simulink model "Final_Simulink_Model_assignment_2"  (R2022b)
settings: Solver=FixedStepAuto  StartTime=0.0  StopTime=inf  FixedStep=1e-3  RelTol=1e-3  EnableMultiTasking=on
undefined symbols (not defined in the file): A0, A1, ATR_PULSE_WIDTH, ATR_PUSLE_WIDTH, D0, D1, D10, D11, D12, D13, D2, D3, D4, D5, D6, D7, D8, D9, LRL, magnitude, PTA0, PTA1, PTA2, PTB2, PTB23, PTB3, PTB9, PTC16, PTC17, PTC2, PTC3, PTC4, PTD0, PTD1, PTD2, PTD3, REF_PERIOD, REF_PREIOD, VENT_PULSE_WIDTH
libraries: frdmk64flib x30, etargetslib x9, dspstat3 x1
(part 2 of 2)

== stateflow chart Final_Simulink_Model_assignment_2/Requirements Table1 ==
  (default) -> (junction 1073743363)
  (junction 1073743363) -> (junction 1073743364) : {
      | % SF_REQ_REV_07
      | }
  (junction 1073743364) -> (junction 1073743366) : {
      | % HEADER_ASSIGNMENTS
      |
      | }
  (junction 1073743366) -> (junction 1073743368) : {
      | % START_A_4
      | }
  (junction 1073743368) -> (junction 1073743370) : {
      | }
  (junction 1073743370) -> (junction 1073743372)
  (junction 1073743372) -> (junction 1073743374) : {
      | }
  (junction 1073743374) -> (junction 1073743376) : {
      | % END_A_4
      | }
  (junction 1073743376) -> (junction 1073743378) : {
      | % START_R_1
      | }
  (junction 1073743378) -> (junction 1073743380) : {
      | }
  (junction 1073743380) -> (junction 1073743382)
  (junction 1073743382) -> (junction 1073743384) [order 1] : [(((Mode) == (1)))]
  (junction 1073743382) -> (junction 1073743426) [order 2]
  (junction 1073743384) -> (junction 1073743386) : {
      |
      |
      | }
  (junction 1073743386) -> (junction 1073743388) : {
      | }
  (junction 1073743388) -> (junction 1073743390) : {
      | % START_R_7
      | }
  (junction 1073743390) -> (junction 1073743392) : {
      | }
  (junction 1073743392) -> (junction 1073743394)
  (junction 1073743394) -> (junction 1073743396) [order 1] : [duration((((State) == (1)))) >= 60000/LRL - ATR_PULSE_WIDTH]
  (junction 1073743394) -> (junction 1073743402) [order 2]
  (junction 1073743396) -> (junction 1073743398) : {
      | reqtable_postcondition((((ATR_PACE_CTRL) == (1))) && (((ATR_GND_CTRL) == (0))) && (((PACE_CHARGE_CTRL) == (0))) && (((PACE_GND_CTRL) == (1))), 'R:1.1');
      |
      |
      | }
  (junction 1073743398) -> (junction 1073743400) : {
      | }
  (junction 1073743400) -> (junction 1073743402)
  (junction 1073743402) -> (junction 1073743404)
  (junction 1073743404) -> (junction 1073743406) : {
      | % END_R_7
      | }
  (junction 1073743406) -> (junction 1073743408) : {
      | % START_R_10
      | }
  (junction 1073743408) -> (junction 1073743410) : {
      | }
  (junction 1073743410) -> (junction 1073743412)
  (junction 1073743412) -> (junction 1073743414) [order 1] : [duration((((State) == (2)))) >= ATR_PULSE_WIDTH]
  (junction 1073743412) -> (junction 1073743420) [order 2]
  (junction 1073743414) -> (junction 1073743416) : {
      | reqtable_postcondition((((ATR_PACE_CTRL) == (0))) && (((ATR_GND_CTRL) == (1))) && (((PACE_CHARGE_CTRL) == (1))) && (((PACE_GND_CTRL) == (1))), 'R:1.2');
      |
      |
      | }
  (junction 1073743416) -> (junction 1073743418) : {
      | }
  (junction 1073743418) -> (junction 1073743420)
  (junction 1073743420) -> (junction 1073743422)
  (junction 1073743422) -> (junction 1073743424) : {
      | % END_R_10
      | }
  (junction 1073743424) -> (junction 1073743426)
  (junction 1073743426) -> (junction 1073743428)
  (junction 1073743428) -> (junction 1073743672) : {
      | % END_R_1
      | }
  (junction 1073743672) -> (junction 1073743432) : {
      | % START_R_13
      | }
  (junction 1073743432) -> (junction 1073743434) : {
      | }
  (junction 1073743434) -> (junction 1073743436)
  (junction 1073743436) -> (junction 1073743438) [order 1] : [(((Mode) == (2)))]
  (junction 1073743436) -> (junction 1073743480) [order 2]
  (junction 1073743438) -> (junction 1073743440) : {
      |
      |
      | }
  (junction 1073743440) -> (junction 1073743442) : {
      | }
  (junction 1073743442) -> (junction 1073743444) : {
      | % START_R_16
      | }
  (junction 1073743444) -> (junction 1073743446) : {
      | }
  (junction 1073743446) -> (junction 1073743448)
  (junction 1073743448) -> (junction 1073743450) [order 1] : [duration((((State) == (1)))) >= 60000/LRL - VENT_PULSE_WIDTH]
  (junction 1073743448) -> (junction 1073743456) [order 2]
  (junction 1073743450) -> (junction 1073743452) : {
      | reqtable_postcondition((((PACE_CHARGE_CTRL) == (0))) && (((PACE_GND_CTRL) == (1))) && (((VENT_PACE_CTRL) == (1))) && (((VENT_GND_CTRL) == (0))), 'R:2.1');
      |
      |
      | }
  (junction 1073743452) -> (junction 1073743454) : {
      | }
  (junction 1073743454) -> (junction 1073743456)
  (junction 1073743456) -> (junction 1073743458)
  (junction 1073743458) -> (junction 1073743460) : {
      | % END_R_16
      | }
  (junction 1073743460) -> (junction 1073743462) : {
      | % START_R_19
      | }
  (junction 1073743462) -> (junction 1073743464) : {
      | }
  (junction 1073743464) -> (junction 1073743466)
  (junction 1073743466) -> (junction 1073743468) [order 1] : [duration((((State) == (2)))) >= VENT_PULSE_WIDTH]
  (junction 1073743466) -> (junction 1073743474) [order 2]
  (junction 1073743468) -> (junction 1073743470) : {
      | reqtable_postcondition((((PACE_CHARGE_CTRL) == (1))) && (((PACE_GND_CTRL) == (1))) && (((VENT_PACE_CTRL) == (0))) && (((VENT_GND_CTRL) == (1))), 'R:2.2');
      |
      |
      | }
  (junction 1073743470) -> (junction 1073743472) : {
      | }
  (junction 1073743472) -> (junction 1073743474)
  (junction 1073743474) -> (junction 1073743476)
  (junction 1073743476) -> (junction 1073743478) : {
      | % END_R_19
      | }
  (junction 1073743478) -> (junction 1073743480)
  (junction 1073743480) -> (junction 1073743482)
  (junction 1073743482) -> (junction 1073743484) : {
      | % END_R_13
      | }
  (junction 1073743484) -> (junction 1073743486) : {
      | % START_R_22
      | }
  (junction 1073743486) -> (junction 1073743488) : {
      | }
  (junction 1073743488) -> (junction 1073743490)
  (junction 1073743490) -> (junction 1073743492) [order 1] : [(((Mode) == (3)))]
  (junction 1073743490) -> (junction 1073743552) [order 2]
  (junction 1073743492) -> (junction 1073743494) : {
      |
      |
      | }
  (junction 1073743494) -> (junction 1073743496) : {
      | }
  (junction 1073743496) -> (junction 1073743498) : {
      | % START_R_25
      | }
  (junction 1073743498) -> (junction 1073743500) : {
      | }
  (junction 1073743500) -> (junction 1073743502)
  (junction 1073743502) -> (junction 1073743504) [order 1] : [duration((((State) == (1)))) >= 60000/LRL - ATR_PULSE_WIDTH]
  (junction 1073743502) -> (junction 1073743510) [order 2]
  (junction 1073743504) -> (junction 1073743506) : {
      | reqtable_postcondition((((ATR_PACE_CTRL) == (0))) && (((ATR_GND_CTRL) == (1))) && (((PACE_CHARGE_CTRL) == (1))) && (((PACE_GND_CTRL) == (1))) && (((FRONTEND_CTRL) == (1))), 'R:3.1');
      |
      |
      | }
  (junction 1073743506) -> (junction 1073743508) : {
      | }
  (junction 1073743508) -> (junction 1073743510)
  (junction 1073743510) -> (junction 1073743512)
  (junction 1073743512) -> (junction 1073743514) : {
      | % END_R_25
      | }
  (junction 1073743514) -> (junction 1073743516) : {
      | % START_R_28
      | }
  (junction 1073743516) -> (junction 1073743518) : {
      | }
  (junction 1073743518) -> (junction 1073743520)
  (junction 1073743520) -> (junction 1073743522) [order 1] : [duration((((State) == (2)))) >= ATR_PULSE_WIDTH]
  (junction 1073743520) -> (junction 1073743528) [order 2]
  (junction 1073743522) -> (junction 1073743524) : {
      | reqtable_postcondition((((ATR_PACE_CTRL) == (1))) && (((ATR_GND_CTRL) == (0))) && (((PACE_CHARGE_CTRL) == (0))) && (((PACE_GND_CTRL) == (1))), 'R:3.2');
      |
      |
      | }
  (junction 1073743524) -> (junction 1073743526) : {
      | }
  (junction 1073743526) -> (junction 1073743528)
  (junction 1073743528) -> (junction 1073743530)
  (junction 1073743530) -> (junction 1073743532) : {
      | % END_R_28
      | }
  (junction 1073743532) -> (junction 1073743534) : {
      | % START_R_31
      | }
  (junction 1073743534) -> (junction 1073743536) : {
      | }
  (junction 1073743536) -> (junction 1073743538)
  (junction 1073743538) -> (junction 1073743540) [order 1] : [duration((((State) == (3)))) >= REF_PERIOD]
  (junction 1073743538) -> (junction 1073743546) [order 2]
  (junction 1073743540) -> (junction 1073743542) : {
      | reqtable_postcondition((((ATR_PACE_CTRL) == (0))) && (((ATR_GND_CTRL) == (1))) && (((PACE_CHARGE_CTRL) == (0))) && (((PACE_GND_CTRL) == (1))) && (((FRONTEND_CTRL) == (0))), 'R:3.3');
      |
      |
      | }
  (junction 1073743542) -> (junction 1073743544) : {
      | }
  (junction 1073743544) -> (junction 1073743546)
  (junction 1073743546) -> (junction 1073743548)
  (junction 1073743548) -> (junction 1073743550) : {
      | % END_R_31
      | }
  (junction 1073743550) -> (junction 1073743552)
  (junction 1073743552) -> (junction 1073743554)
  (junction 1073743554) -> (junction 1073743556) : {
      | % END_R_22
      | }
  (junction 1073743556) -> (junction 1073743558) : {
      | % START_R_34
      | }
  (junction 1073743558) -> (junction 1073743560) : {
      | }
  (junction 1073743560) -> (junction 1073743562)
  (junction 1073743562) -> (junction 1073743564) [order 1] : [(((Mode) == (4)))]
  (junction 1073743562) -> (junction 1073743624) [order 2]
  (junction 1073743564) -> (junction 1073743566) : {
      |
      |
      | }
  (junction 1073743566) -> (junction 1073743568) : {
      | }
  (junction 1073743568) -> (junction 1073743570) : {
      | % START_R_37
      | }
  (junction 1073743570) -> (junction 1073743572) : {
      | }
  (junction 1073743572) -> (junction 1073743574)
  (junction 1073743574) -> (junction 1073743576) [order 1] : [duration((((State) == (1)))) >= 60000/LRL - VENT_PULSE_WIDTH]
  (junction 1073743574) -> (junction 1073743582) [order 2]
  (junction 1073743576) -> (junction 1073743578) : {
      | reqtable_postcondition((((PACE_CHARGE_CTRL) == (1))) && (((PACE_GND_CTRL) == (1))) && (((VENT_PACE_CTRL) == (0))) && (((VENT_GND_CTRL) == (1))) && (((FRONTEND_CTRL) == (1))), 'R:4.1');
      |
      |
      | }
  (junction 1073743578) -> (junction 1073743580) : {
      | }
  (junction 1073743580) -> (junction 1073743582)
  (junction 1073743582) -> (junction 1073743584)
  (junction 1073743584) -> (junction 1073743586) : {
      | % END_R_37
      | }
  (junction 1073743586) -> (junction 1073743588) : {
      | % START_R_40
      | }
  (junction 1073743588) -> (junction 1073743590) : {
      | }
  (junction 1073743590) -> (junction 1073743592)
  (junction 1073743592) -> (junction 1073743594) [order 1] : [duration((((State) == (2)))) >= VENT_PULSE_WIDTH]
  (junction 1073743592) -> (junction 1073743600) [order 2]
  (junction 1073743594) -> (junction 1073743596) : {
      | reqtable_postcondition((((PACE_CHARGE_CTRL) == (0))) && (((PACE_GND_CTRL) == (1))) && (((VENT_PACE_CTRL) == (1))) && (((VENT_GND_CTRL) == (0))), 'R:4.2');
      |
      |
      | }
  (junction 1073743596) -> (junction 1073743598) : {
      | }
  (junction 1073743598) -> (junction 1073743600)
  (junction 1073743600) -> (junction 1073743602)
  (junction 1073743602) -> (junction 1073743604) : {
      | % END_R_40
      | }
  (junction 1073743604) -> (junction 1073743606) : {
      | % START_R_43
      | }
  (junction 1073743606) -> (junction 1073743608) : {
      | }
  (junction 1073743608) -> (junction 1073743610)
  (junction 1073743610) -> (junction 1073743612) [order 1] : [duration((((State) == (3)))) >= REF_PREIOD]
  (junction 1073743610) -> (junction 1073743618) [order 2]
  (junction 1073743612) -> (junction 1073743614) : {
      | reqtable_postcondition((((PACE_CHARGE_CTRL) == (0))) && (((PACE_GND_CTRL) == (1))) && (((VENT_PACE_CTRL) == (0))) && (((VENT_GND_CTRL) == (1))) && (((FRONTEND_CTRL) == (0))), 'R:4.3');
      |
      |
      | }
  (junction 1073743614) -> (junction 1073743616) : {
      | }
  (junction 1073743616) -> (junction 1073743618)
  (junction 1073743618) -> (junction 1073743620)
  (junction 1073743620) -> (junction 1073743660) : {
      | % END_R_43
      | }
  (junction 1073743660) -> (junction 1073743624)
  (junction 1073743624) -> (junction 1073743626)
  (junction 1073743626) -> (junction 1073743628) : {
      | % END_R_34
      | }
  (junction 1073743628) -> (junction 1073743709) : {
      | % START_R_46
      | }
  (junction 1073743709) -> (junction 1073743711) : {
      | }
  (junction 1073743711) -> (junction 1073743713)
  (junction 1073743713) -> (junction 1073743715) [order 1] : [(((Mode) == (5)))]
  (junction 1073743713) -> (junction 1073743731) [order 2]
  (junction 1073743715) -> (junction 1073743717) : {
      |
      |
      | }
  (junction 1073743717) -> (junction 1073743719) : {
      | }
  (junction 1073743719) -> (junction 1073743786) : {
      | % START_R_49
      | }
  (junction 1073743786) -> (junction 1073743788) : {
      | }
  (junction 1073743788) -> (junction 1073743790)
  (junction 1073743790) -> (junction 1073743792) [order 1] : [duration((((State) == (1)))) >= 60000/Rate-ATR_PULSE_WIDTH]
  (junction 1073743790) -> (junction 1073743798) [order 2]
  (junction 1073743792) -> (junction 1073743794) : {
      | reqtable_postcondition((((ATR_PACE_CTRL) == (1))) && (((ATR_GND_CTRL) == (0))) && (((PACE_CHARGE_CTRL) == (0))) && (((PACE_GND_CTRL) == (1))), 'R:5.1');
      |
      |
      | }
  (junction 1073743794) -> (junction 1073743796) : {
      | }
  (junction 1073743796) -> (junction 1073743798)
  (junction 1073743798) -> (junction 1073743800)
  (junction 1073743800) -> (junction 1073743802) : {
      | % END_R_49
      | }
  (junction 1073743802) -> (junction 1073743807) : {
      | % START_R_52
      | }
  (junction 1073743807) -> (junction 1073743809) : {
      | }
  (junction 1073743809) -> (junction 1073743811)
  (junction 1073743811) -> (junction 1073743813) [order 1] : [duration((((State) == (2)))) >= ATR_PULSE_WIDTH]
  (junction 1073743811) -> (junction 1073743819) [order 2]
  (junction 1073743813) -> (junction 1073743815) : {
      | reqtable_postcondition((((ATR_PACE_CTRL) == (0))) && (((ATR_GND_CTRL) == (1))) && (((PACE_CHARGE_CTRL) == (1))) && (((PACE_GND_CTRL) == (1))), 'R:5.2');
      |
      |
      | }
  (junction 1073743815) -> (junction 1073743817) : {
      | }
  (junction 1073743817) -> (junction 1073743819)
  (junction 1073743819) -> (junction 1073743821)
  (junction 1073743821) -> (junction 1073743823) : {
      | % END_R_52
      | }
  (junction 1073743823) -> (junction 1073743731)
  (junction 1073743731) -> (junction 1073743733)
  (junction 1073743733) -> (junction 1073743735) : {
      | % END_R_46
      | }
  (junction 1073743735) -> (junction 1073743974) : {
      | % START_R_55
      | }
  (junction 1073743974) -> (junction 1073743976) : {
      | }
  (junction 1073743976) -> (junction 1073743978)
  (junction 1073743978) -> (junction 1073743980) [order 1] : [(((Mode) == (6)))]
  (junction 1073743978) -> (junction 1073744022) [order 2]
  (junction 1073743980) -> (junction 1073743982) : {
      |
      |
      | }
  (junction 1073743982) -> (junction 1073743984) : {
      | }
  (junction 1073743984) -> (junction 1073743986) : {
      | % START_R_58
      | }
  (junction 1073743986) -> (junction 1073743988) : {
      | }
  (junction 1073743988) -> (junction 1073743990)
  (junction 1073743990) -> (junction 1073743992) [order 1] : [duration((((State) == (1)))) >= 60000/ Rate- VENT_PULSE_WIDTH]
  (junction 1073743990) -> (junction 1073743998) [order 2]
  (junction 1073743992) -> (junction 1073743994) : {
      | reqtable_postcondition((((PACE_CHARGE_CTRL) == (0))) && (((PACE_GND_CTRL) == (1))) && (((VENT_PACE_CTRL) == (1))) && (((VENT_GND_CTRL) == (0))), 'R:6.1');
      |
      |
      | }
  (junction 1073743994) -> (junction 1073743996) : {
      | }
  (junction 1073743996) -> (junction 1073743998)
  (junction 1073743998) -> (junction 1073744000)
  (junction 1073744000) -> (junction 1073744002) : {
      | % END_R_58
      | }
  (junction 1073744002) -> (junction 1073744004) : {
      | % START_R_61
      | }
  (junction 1073744004) -> (junction 1073744006) : {
      | }
  (junction 1073744006) -> (junction 1073744008)
  (junction 1073744008) -> (junction 1073744010) [order 1] : [duration((((State) == (2)))) >= VENT_PULSE_WIDTH]
  (junction 1073744008) -> (junction 1073744016) [order 2]
  (junction 1073744010) -> (junction 1073744012) : {
      | reqtable_postcondition((((PACE_CHARGE_CTRL) == (1))) && (((PACE_GND_CTRL) == (1))) && (((VENT_PACE_CTRL) == (0))) && (((VENT_GND_CTRL) == (1))), 'R:6.2');
      |
      |
      | }
  (junction 1073744012) -> (junction 1073744014) : {
      | }
  (junction 1073744014) -> (junction 1073744016)
  (junction 1073744016) -> (junction 1073744018)
  (junction 1073744018) -> (junction 1073744020) : {
      | % END_R_61
      | }
  (junction 1073744020) -> (junction 1073744022)
  (junction 1073744022) -> (junction 1073744024)
  (junction 1073744024) -> (junction 1073744026) : {
      | % END_R_55
      | }
  (junction 1073744026) -> (junction 1073744033) : {
      | % START_R_64
      | }
  (junction 1073744033) -> (junction 1073744035) : {
      | }
  (junction 1073744035) -> (junction 1073744037)
  (junction 1073744037) -> (junction 1073744039) [order 1] : [(((Mode) == (7)))]
  (junction 1073744037) -> (junction 1073744075) [order 2]
  (junction 1073744039) -> (junction 1073744041) : {
      |
      |
      | }
  (junction 1073744041) -> (junction 1073744043) : {
      | }
  (junction 1073744043) -> (junction 1073744084) : {
      | % START_R_67
      | }
  (junction 1073744084) -> (junction 1073744086) : {
      | }
  (junction 1073744086) -> (junction 1073744088)
  (junction 1073744088) -> (junction 1073744090) [order 1] : [duration((((State) == (1)))) >= 60000/Rate-ATR_PULSE_WIDTH-ARP]
  (junction 1073744088) -> (junction 1073744096) [order 2]
  (junction 1073744090) -> (junction 1073744092) : {
      | reqtable_postcondition((((ATR_PACE_CTRL) == (0))) && (((ATR_GND_CTRL) == (1))) && (((PACE_CHARGE_CTRL) == (1))) && (((PACE_GND_CTRL) == (1))) && (((FRONTEND_CTRL) == (1))), 'R:7.1');
      |
      |
      | }
  (junction 1073744092) -> (junction 1073744094) : {
      | }
  (junction 1073744094) -> (junction 1073744096)
  (junction 1073744096) -> (junction 1073744098)
  (junction 1073744098) -> (junction 1073744100) : {
      | % END_R_67
      | }
  (junction 1073744100) -> (junction 1073744105) : {
      | % START_R_70
      | }
  (junction 1073744105) -> (junction 1073744107) : {
      | }
  (junction 1073744107) -> (junction 1073744109)
  (junction 1073744109) -> (junction 1073744111) [order 1] : [duration((((State) == (2)))) >= ARP]
  (junction 1073744109) -> (junction 1073744117) [order 2]
  (junction 1073744111) -> (junction 1073744113) : {
      | reqtable_postcondition((((ATR_PACE_CTRL) == (1))) && (((ATR_GND_CTRL) == (0))) && (((PACE_CHARGE_CTRL) == (0))) && (((PACE_GND_CTRL) == (1))), 'R:7.2');
      |
      |
      | }
  (junction 1073744113) -> (junction 1073744115) : {
      | }
  (junction 1073744115) -> (junction 1073744117)
  (junction 1073744117) -> (junction 1073744119)
  (junction 1073744119) -> (junction 1073744121) : {
      | % END_R_70
      | }
  (junction 1073744121) -> (junction 1073744126) : {
      | % START_R_73
      | }
  (junction 1073744126) -> (junction 1073744128) : {
      | }
  (junction 1073744128) -> (junction 1073744130)
  (junction 1073744130) -> (junction 1073744132) [order 1] : [duration((((State) == (3)))) >= ARP]
  (junction 1073744130) -> (junction 1073744138) [order 2]
  (junction 1073744132) -> (junction 1073744134) : {
      | reqtable_postcondition((((ATR_PACE_CTRL) == (0))) && (((ATR_GND_CTRL) == (1))) && (((PACE_CHARGE_CTRL) == (0))) && (((PACE_GND_CTRL) == (1))) && (((FRONTEND_CTRL) == (0))), 'R:7.3');
      |
      |
      | }
  (junction 1073744134) -> (junction 1073744136) : {
      | }
  (junction 1073744136) -> (junction 1073744138)
  (junction 1073744138) -> (junction 1073744140)
  (junction 1073744140) -> (junction 1073744142) : {
      | % END_R_73
      | }
  (junction 1073744142) -> (junction 1073744075)
  (junction 1073744075) -> (junction 1073744077)
  (junction 1073744077) -> (junction 1073744079) : {
      | % END_R_64
      | }
  (junction 1073744079) -> (junction 1073744180) : {
      | % START_R_76
      | }
  (junction 1073744180) -> (junction 1073744182) : {
      | }
  (junction 1073744182) -> (junction 1073744184)
  (junction 1073744184) -> (junction 1073744186) [order 1] : [(((Mode) == (8)))]
  (junction 1073744184) -> (junction 1073744202) [order 2]
  (junction 1073744186) -> (junction 1073744188) : {
      |
      |
      | }
  (junction 1073744188) -> (junction 1073744190) : {
      | }
  (junction 1073744190) -> (junction 1073744269) : {
      | % START_R_79
      | }
  (junction 1073744269) -> (junction 1073744271) : {
      | }
  (junction 1073744271) -> (junction 1073744273)
  (junction 1073744273) -> (junction 1073744275) [order 1] : [duration((((State) == (1)))) >= 60000/Rate-VENT_PULSE_WIDTH-VRP]
  (junction 1073744273) -> (junction 1073744281) [order 2]
  (junction 1073744275) -> (junction 1073744277) : {
      | reqtable_postcondition((((PACE_CHARGE_CTRL) == (1))) && (((PACE_GND_CTRL) == (1))) && (((VENT_PACE_CTRL) == (0))) && (((VENT_GND_CTRL) == (1))) && (((FRONTEND_CTRL) == (1))), 'R:8.1');
      |
      |
      | }
  (junction 1073744277) -> (junction 1073744279) : {
      | }
  (junction 1073744279) -> (junction 1073744281)
  (junction 1073744281) -> (junction 1073744283)
  (junction 1073744283) -> (junction 1073744285) : {
      | % END_R_79
      | }
  (junction 1073744285) -> (junction 1073744290) : {
      | % START_R_85
      | }
  (junction 1073744290) -> (junction 1073744292) : {
      | }
  (junction 1073744292) -> (junction 1073744294)
  (junction 1073744294) -> (junction 1073744296) [order 1] : [duration((((State) == (2)))) >= VRP]
  (junction 1073744294) -> (junction 1073744302) [order 2]
  (junction 1073744296) -> (junction 1073744298) : {
      | reqtable_postcondition((((PACE_CHARGE_CTRL) == (0))) && (((PACE_GND_CTRL) == (1))) && (((VENT_PACE_CTRL) == (1))) && (((VENT_GND_CTRL) == (0))), 'R:8.2');
      |
      |
      | }
  (junction 1073744298) -> (junction 1073744300) : {
      | }
  (junction 1073744300) -> (junction 1073744302)
  (junction 1073744302) -> (junction 1073744304)
  (junction 1073744304) -> (junction 1073744306) : {
      | % END_R_85
      | }
  (junction 1073744306) -> (junction 1073744311) : {
      | % START_R_88
      | }
  (junction 1073744311) -> (junction 1073744313) : {
      | }
  (junction 1073744313) -> (junction 1073744315)
  (junction 1073744315) -> (junction 1073744317) [order 1] : [duration((((State) == (3)))) >= VRP]
  (junction 1073744315) -> (junction 1073744323) [order 2]
  (junction 1073744317) -> (junction 1073744319) : {
      | reqtable_postcondition((((PACE_CHARGE_CTRL) == (0))) && (((PACE_GND_CTRL) == (1))) && (((VENT_GND_CTRL) == (1))) && (((FRONTEND_CTRL) == (0))), 'R:8.3');
      |
      |
      | }
  (junction 1073744319) -> (junction 1073744321) : {
      | }
  (junction 1073744321) -> (junction 1073744323)
  (junction 1073744323) -> (junction 1073744325)
  (junction 1073744325) -> (junction 1073744327) : {
      | % END_R_88
      | }
  (junction 1073744327) -> (junction 1073744202)
  (junction 1073744202) -> (junction 1073744204)
  (junction 1073744204) -> (junction 1073744206) : {
      | % END_R_76
      | }
  data: State input; FRONTEND_CTRL input; VENT_PACE_CTRL input; VENT_GND_CTRL input; ATR_PACE_CTRL input; ATR_GND_CTRL input; PACE_CHARGE_CTRL input; PACE_GND_CTRL input; Mode input double; VENT_CMP_DETECT input; ATR_CMP_DETECT input; ATR_PULSE_WIDTH parameter; LRL parameter; ATR_PUSLE_WIDTH parameter; VENT_PULSE_WIDTH parameter; REF_PREIOD parameter; REF_PERIOD parameter
